simulink model "Simulink_Model"  (R2022a)
settings: Solver=VariableStepAuto  StartTime=0.0  StopTime=2474  RelTol=1e-3
values from neighbouring files (symbols this model uses):
  Air_Density = 1.2    [car__specifications.mat]
  Angle = 0    [car__specifications.mat]
  Battery_Cell_Volume = 16532.1    [car__specifications.mat]
  Battery_Cell_Weight = 0.05    [car__specifications.mat]
  constant = 0.10471975512    [car__specifications.mat]
  Drag_Coefficient = 0.2    [car__specifications.mat]
  Frontal_Area = 2.65    [car__specifications.mat]
  Gear_Ratio = 9    [car__specifications.mat]
  Motor_Efficiency = 0.95    [car__specifications.mat]
  Nominal_Battery_Cell_Current_Rating = 2.5    [car__specifications.mat]
  Nominal_Battery_Cell_Voltage = 3.6    [car__specifications.mat]
  Nominal_Battery_Pack_Voltage = 220    [car__specifications.mat]
  Range = 300    [car__specifications.mat]
  Rolling_Resistance_Coefficient = 0.02    [car__specifications.mat]
  Transmission_Efficiency = 0.8    [car__specifications.mat]
  Vehicle_Mass = 1000    [car__specifications.mat]
  Wheel_Radius = 0.3    [car__specifications.mat]
libraries: autolibshared x1
settings Model: Creator=jamesbond  LastModifiedBy=jamesbond

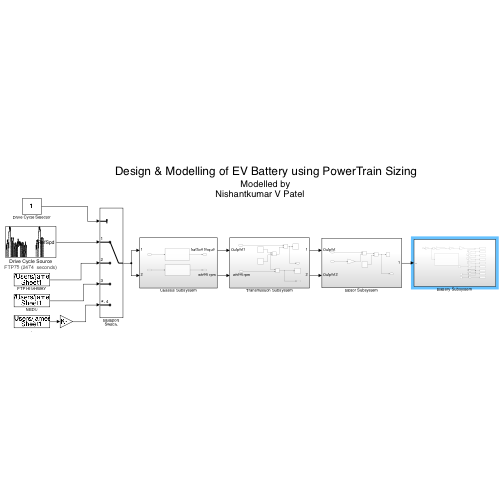
[thumbnail: Simulink's stored preview of the top-level diagram]
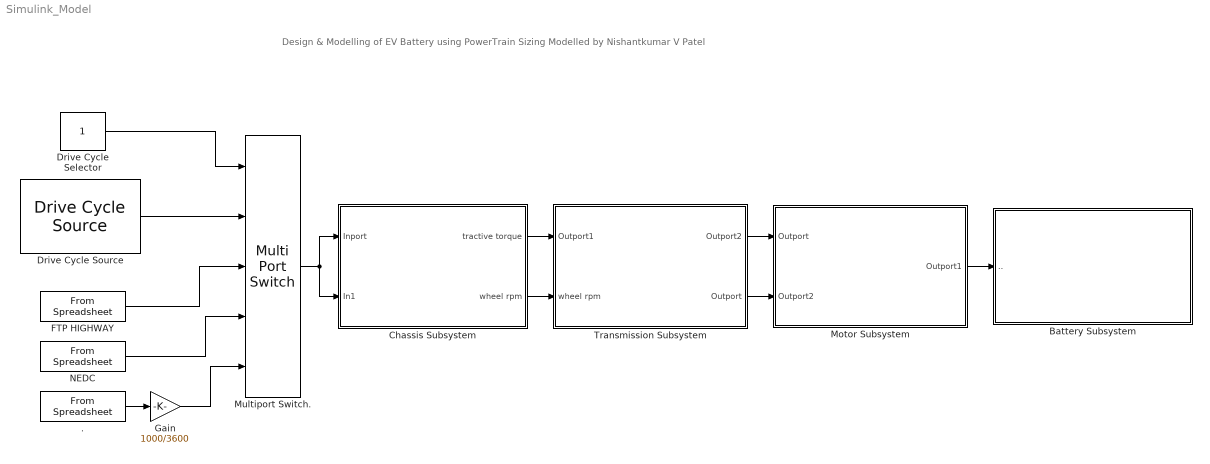
== system Simulink_Model ==
  note: Design & Modelling of EV Battery using PowerTrain Sizing
      | Modelled by
      | Nishantkumar V Patel
  . : FromSpreadsheet  FileName=/Users/jamesbond/Desktop/Mathematical Modelling of Physical Systems/Modelling & Designing EV Battery using PowerTrain Sizing Calculations /Drive Cycle Excel Files/WLTP.xlsx
  Battery Subsystem : Subsystem
  Chassis Subsystem : Subsystem
  Drive Cycle Selector : Constant
  Drive Cycle Source : autolibshared/Drive Cycle Source  cycleVar=FTP75  fileVar=WLTP.xlss  tfinal="2474  seconds"  cycleRepeat=off  outAccPort=off  outGearPort=off  gearList=No gear data  t_wot1=5  xdot_woto=0  xdot_wot1=30  t_wot2=20  xdot_wot2=0  t_wotend=30  srcUnit=m/s  outUnit=m/s  srcAccUnit=m/s/s  outAccUnit=m/s^2  dt=0  aMode=1  faultOption=off  velBnd=2  velBndUnit=mph  inUnit=m/s  timeBnd=1  failOption=off  stopSim=off  maxFaultCnt=10  maxFaultTime=2  maxTotFaultTime=15  traceOption=off  dtTrace=1  traceWindow=10  lastDCname=FTP75  lastOutUnit=mph  lastDT=0  lastTB=1  lastSB=2  forceCalcBound=off
      settings: SourceProductBaseCode=PW,DR,MT,VE
  FTP HIGHWAY : FromSpreadsheet  FileName=/Users/jamesbond/Desktop/Mathematical Modelling of Physical Systems/Modelling & Designing EV Battery using PowerTrain Sizing Calculations /Drive Cycle Excel Files/FTP_HIGHWAY.xlsx
  Gain : Gain  Gain=1000/3600
  Motor Subsystem : Subsystem
  Multiport Switch. : MultiPortSwitch  Inputs=4  SaturateOnIntegerOverflow=off  InputSameDT=off
  NEDC : FromSpreadsheet  FileName=/Users/jamesbond/Desktop/Mathematical Modelling of Physical Systems/Modelling & Designing EV Battery using PowerTrain Sizing Calculations /Drive Cycle Excel Files/NEDC.xlsx
  Transmission Subsystem : Subsystem
  wires:
  Drive Cycle Selector/1 -> Multiport Switch./1
  Drive Cycle Source/1 -> Multiport Switch./2
  FTP HIGHWAY/1 -> Multiport Switch./3
  NEDC/1 -> Multiport Switch./4
  ./1 -> Gain/1
  Gain/1 -> Multiport Switch./5
  Multiport Switch./1 -> Chassis Subsystem/1(Inport), Chassis Subsystem/2(In1)
  Motor Subsystem/1(Outport1) -> Battery Subsystem/1(..)
  Chassis Subsystem/2("  wheel rpm") -> Transmission Subsystem/2("  wheel rpm")
  Chassis Subsystem/1("tractive torque ") -> Transmission Subsystem/1(Outport1)
  Transmission Subsystem/1(Outport2) -> Motor Subsystem/1(Outport)
  Transmission Subsystem/2(Outport) -> Motor Subsystem/2(Outport2)

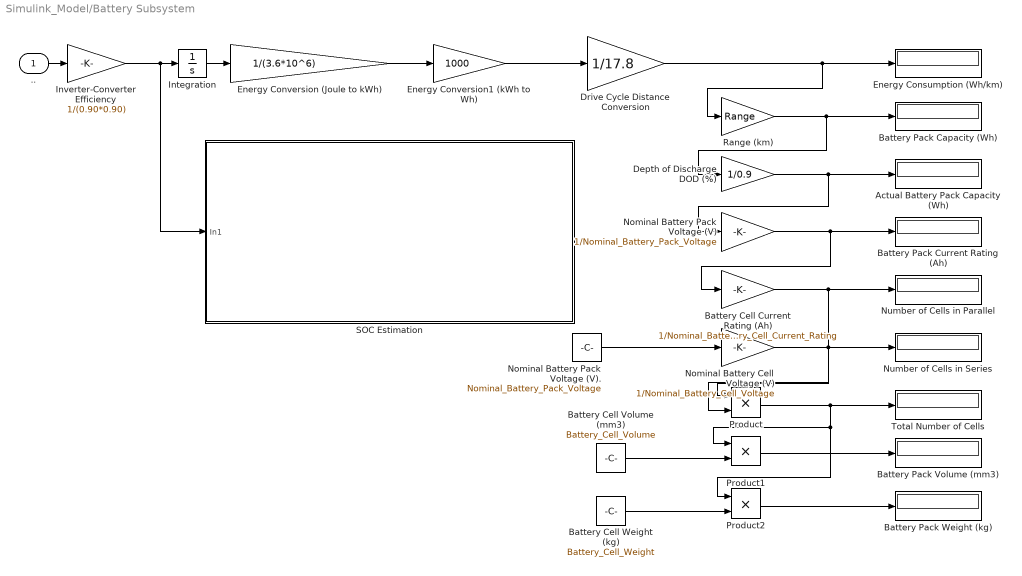
== system Simulink_Model/Battery Subsystem ==
  .. : Inport
  Actual Battery Pack Capacity (Wh) : Display
  Battery Cell Current Rating (Ah) : Gain  Gain=1/Nominal_Battery_Cell_Current_Rating
  Battery Cell Volume (mm3) : Constant  Value=Battery_Cell_Volume
  Battery Cell Weight (kg) : Constant  Value=Battery_Cell_Weight
  Battery Pack Capacity (Wh) : Display
  Battery Pack Current Rating (Ah) : Display
  Battery Pack Volume (mm3) : Display
  Battery Pack Weight (kg) : Display
  Depth of Discharge DOD (%) : Gain  Gain=1/0.9
  Drive Cycle Distance Conversion : Gain  Gain=1/17.8
  Energy Consumption (Wh/km) : Display
  "Energy Conversion (Joule to kWh) " : Gain  Gain=1/(3.6*10^6)
  Energy Conversion1 (kWh to Wh) : Gain  Gain=1000
  Integration : Integrator
  Inverter-Converter Efficiency : Gain  Gain=1/(0.90*0.90)
  Nominal Battery Cell Voltage (V) : Gain  Gain=1/Nominal_Battery_Cell_Voltage
  Nominal Battery Pack Voltage (V) : Gain  Gain=1/Nominal_Battery_Pack_Voltage
  Nominal Battery Pack Voltage (V). : Constant  Value=Nominal_Battery_Pack_Voltage
  Number of Cells in Parallel : Display
  Number of Cells in Series : Display
  Product : Product
  Product1 : Product
  Product2 : Product
  Range (km) : Gain  Gain=Range
  SOC Estimation : Subsystem
  Total Number of Cells : Display
  wires:
  ../1 -> Inverter-Converter Efficiency/1
  Inverter-Converter Efficiency/1 -> SOC Estimation/1(In1), Integration/1
  Integration/1 -> "Energy Conversion (Joule to kWh) "/1
  "Energy Conversion (Joule to kWh) "/1 -> Energy Conversion1 (kWh to Wh)/1
  Energy Conversion1 (kWh to Wh)/1 -> Drive Cycle Distance Conversion/1
  Drive Cycle Distance Conversion/1 -> Energy Consumption (Wh/km)/1, Range (km)/1
  Range (km)/1 -> Battery Pack Capacity (Wh)/1, Depth of Discharge DOD (%)/1
  Depth of Discharge DOD (%)/1 -> Actual Battery Pack Capacity (Wh)/1, Nominal Battery Pack Voltage (V)/1
  Nominal Battery Pack Voltage (V)/1 -> Battery Cell Current Rating (Ah)/1, Battery Pack Current Rating (Ah)/1
  Battery Cell Current Rating (Ah)/1 -> Number of Cells in Parallel/1, Product/1
  Nominal Battery Pack Voltage (V)./1 -> Nominal Battery Cell Voltage (V)/1
  Nominal Battery Cell Voltage (V)/1 -> Number of Cells in Series/1, Product/2
  Product/1 -> Product1/1, Product2/1, Total Number of Cells/1
  Product1/1 -> Battery Pack Volume (mm3)/1
  Battery Cell Volume (mm3)/1 -> Product1/2
  Product2/1 -> Battery Pack Weight (kg)/1
  Battery Cell Weight (kg)/1 -> Product2/2

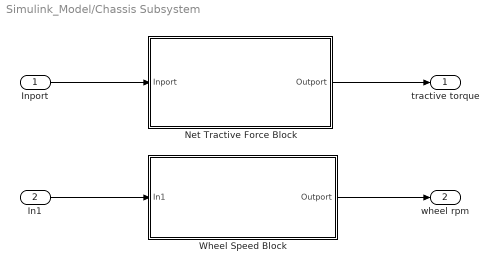
== system Simulink_Model/Chassis Subsystem ==
  Inport : Inport
  In1 : Inport  Port=2
  Net Tractive Force Block : Subsystem
  Wheel Speed Block : Subsystem
  "tractive torque " : Outport
  "  wheel rpm" : Outport  Port=2
  wires:
  Net Tractive Force Block/1(Outport) -> "tractive torque "/1
  Inport/1 -> Net Tractive Force Block/1(Inport)
  In1/1 -> Wheel Speed Block/1(In1)
  Wheel Speed Block/1(Outport) -> "  wheel rpm"/1

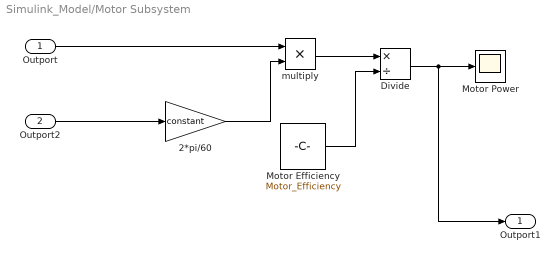
== system Simulink_Model/Motor Subsystem ==
  Outport : Inport
  Outport2 : Inport  Port=2
  2*pi/60 : Gain  Gain=constant
  Divide : Product  Inputs=*/
  Motor Efficiency : Constant  Value=Motor_Efficiency
  Motor Power : Scope
  multiply : Product
  Outport1 : Outport
  wires:
  Outport/1 -> multiply/1
  multiply/1 -> Divide/1
  Motor Efficiency/1 -> Divide/2
  2*pi/60/1 -> multiply/2
  Outport2/1 -> 2*pi/60/1
  Divide/1 -> Outport1/1, Motor Power/1

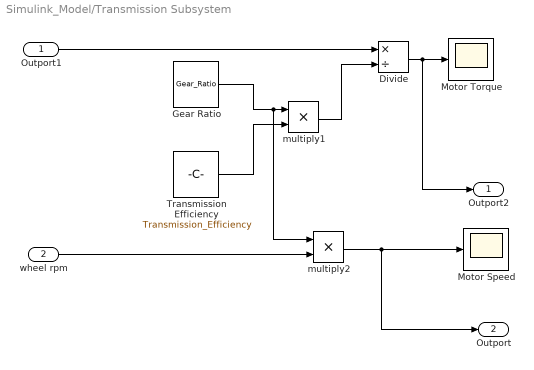
== system Simulink_Model/Transmission Subsystem ==
  Outport1 : Inport
  "  wheel rpm" : Inport  Port=2
  Divide : Product  Inputs=*/
  Gear Ratio : Constant  Value=Gear_Ratio
  Motor Speed : Scope
  Motor Torque : Scope
  Transmission Efficiency : Constant  Value=Transmission_Efficiency
  multiply1 : Product
  multiply2 : Product
  Outport2 : Outport
  Outport : Outport  Port=2
  wires:
  "  wheel rpm"/1 -> multiply2/2
  Divide/1 -> Outport2/1, Motor Torque/1
  multiply2/1 -> Outport/1, Motor Speed/1
  multiply1/1 -> Divide/2
  Outport1/1 -> Divide/1
  Transmission Efficiency/1 -> multiply1/2
  Gear Ratio/1 -> multiply2/1, multiply1/1

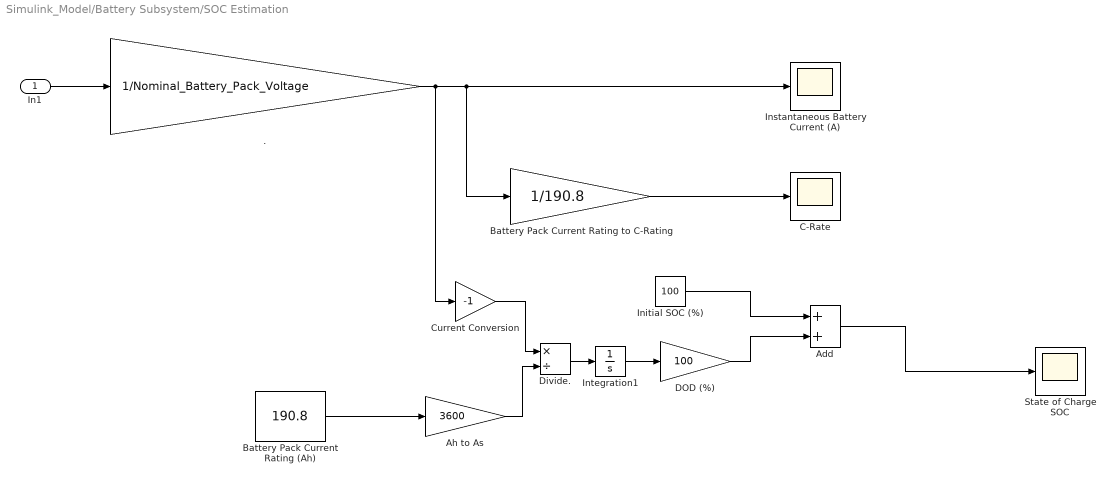
== system Simulink_Model/Battery Subsystem/SOC Estimation ==
  In1 : Inport
  . : Gain  Gain=1/Nominal_Battery_Pack_Voltage
  Add : Sum
  Ah to As : Gain  Gain=3600
  "Battery Pack Current Rating (Ah) " : Constant  Value=190.8
  Battery Pack Current Rating to C-Rating : Gain  Gain=1/190.8
  C-Rate : Scope
  Current Conversion : Gain  Gain=-1
  DOD (%) : Gain  Gain=100
  "Divide. " : Product  Inputs=*/
  Initial SOC (%) : Constant  Value=100
  Instantaneous Battery Current (A) : Scope
  Integration1 : Integrator
  State of Charge SOC : Scope
  wires:
  Add/1 -> State of Charge SOC/1
  "Battery Pack Current Rating (Ah) "/1 -> Ah to As/1
  DOD (%)/1 -> Add/2
  Current Conversion/1 -> "Divide. "/1
  "Divide. "/1 -> Integration1/1
  Initial SOC (%)/1 -> Add/1
  Integration1/1 -> DOD (%)/1
  ./1 -> Current Conversion/1, Battery Pack Current Rating to C-Rating/1, Instantaneous Battery Current (A)/1
  Battery Pack Current Rating to C-Rating/1 -> C-Rate/1
  In1/1 -> ./1
  Ah to As/1 -> "Divide. "/2

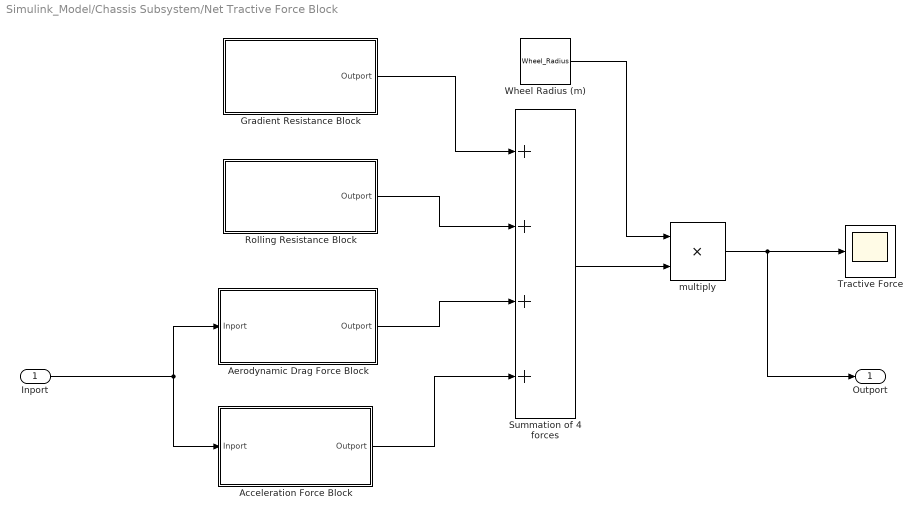
== system Simulink_Model/Chassis Subsystem/Net Tractive Force Block ==
  Inport : Inport
  Acceleration Force Block : Subsystem
  Aerodynamic Drag Force Block : Subsystem
  Gradient Resistance Block : Subsystem
  Rolling Resistance Block : Subsystem
  Summation of 4 forces : Sum  Inputs=++++
  Tractive Force : Scope
  Wheel Radius (m) : Constant  Value=Wheel_Radius
  multiply : Product
  Outport : Outport
  wires:
  Inport/1 -> Acceleration Force Block/1(Inport), Aerodynamic Drag Force Block/1(Inport)
  Gradient Resistance Block/1(Outport) -> Summation of 4 forces/1
  Aerodynamic Drag Force Block/1(Outport) -> Summation of 4 forces/3
  Rolling Resistance Block/1(Outport) -> Summation of 4 forces/2
  Acceleration Force Block/1(Outport) -> Summation of 4 forces/4
  Summation of 4 forces/1 -> multiply/2
  Wheel Radius (m)/1 -> multiply/1
  multiply/1 -> Tractive Force/1, Outport/1

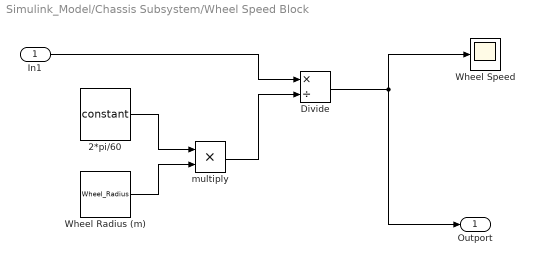
== system Simulink_Model/Chassis Subsystem/Wheel Speed Block ==
  In1 : Inport
  2*pi/60 : Constant  Value=constant
  Divide : Product  Inputs=*/
  Wheel Radius (m) : Constant  Value=Wheel_Radius
  Wheel Speed : Scope
  multiply : Product
  Outport : Outport
  wires:
  In1/1 -> Divide/1
  Wheel Radius (m)/1 -> multiply/2
  2*pi/60/1 -> multiply/1
  Divide/1 -> Wheel Speed/1, Outport/1
  multiply/1 -> Divide/2

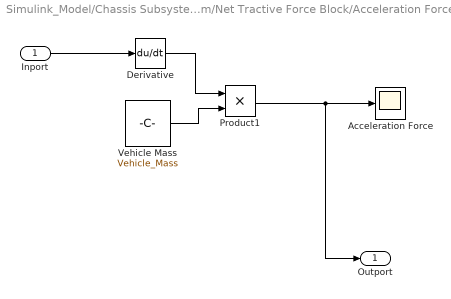
== system Simulink_Model/Chassis Subsystem/Net Tractive Force Block/Acceleration Force Block ==
  Inport : Inport
  Acceleration Force : Scope
  Derivative : Derivative
  Product1 : Product
  Vehicle Mass : Constant  Value=Vehicle_Mass
  Outport : Outport
  wires:
  Vehicle Mass/1 -> Product1/2
  Inport/1 -> Derivative/1
  Derivative/1 -> Product1/1
  Product1/1 -> Outport/1, Acceleration Force/1

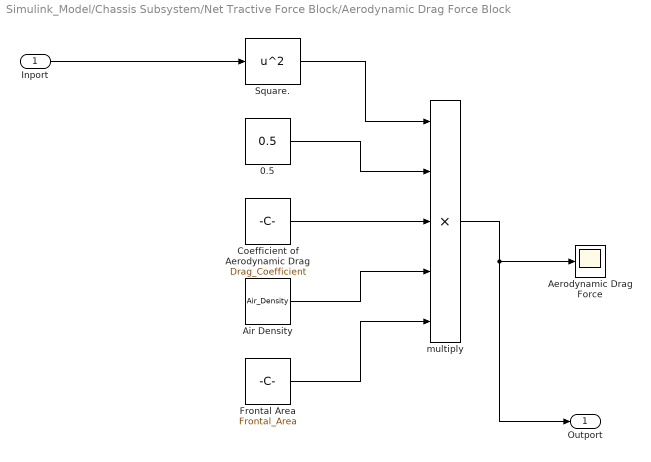
== system Simulink_Model/Chassis Subsystem/Net Tractive Force Block/Aerodynamic Drag Force Block ==
  Inport : Inport
  0.5 : Constant  Value=0.5
  Aerodynamic Drag Force : Scope
  Air Density : Constant  Value=Air_Density
  Coefficient of Aerodynamic Drag : Constant  Value=Drag_Coefficient
  Frontal Area : Constant  Value=Frontal_Area
  Square. : Math  Operator=square
  multiply : Product  Inputs=5
  Outport : Outport
  wires:
  multiply/1 -> Outport/1, Aerodynamic Drag Force/1
  Square./1 -> multiply/1
  0.5/1 -> multiply/2
  Coefficient of Aerodynamic Drag/1 -> multiply/3
  Air Density/1 -> multiply/4
  Frontal Area/1 -> multiply/5
  Inport/1 -> Square./1

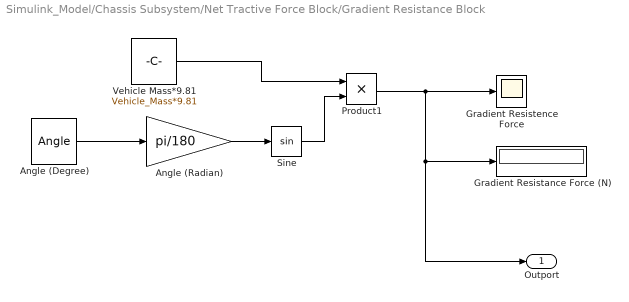
== system Simulink_Model/Chassis Subsystem/Net Tractive Force Block/Gradient Resistance Block ==
  Angle (Degree) : Constant  Value=Angle
  Angle (Radian) : Gain  Gain=pi/180
  Gradient Resistance Force (N) : Display
  Gradient Resistence Force : Scope
  Product1 : Product
  Sine : Trigonometry
  Vehicle Mass*9.81 : Constant  Value=Vehicle_Mass*9.81
  Outport : Outport
  wires:
  Angle (Radian)/1 -> Sine/1
  Sine/1 -> Product1/2
  Vehicle Mass*9.81/1 -> Product1/1
  Product1/1 -> Gradient Resistance Force (N)/1, Outport/1, Gradient Resistence Force/1
  Angle (Degree)/1 -> Angle (Radian)/1

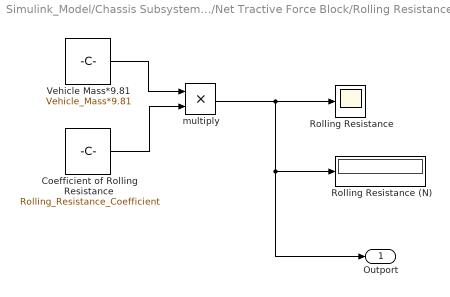
== system Simulink_Model/Chassis Subsystem/Net Tractive Force Block/Rolling Resistance Block ==
  Coefficient of Rolling Resistance : Constant  Value=Rolling_Resistance_Coefficient
  Rolling Resistance : Scope
  Rolling Resistance (N) : Display
  Vehicle Mass*9.81 : Constant  Value=Vehicle_Mass*9.81
  multiply : Product
  Outport : Outport
  wires:
  Vehicle Mass*9.81/1 -> multiply/1
  Coefficient of Rolling Resistance/1 -> multiply/2
  multiply/1 -> Rolling Resistance/1, Rolling Resistance (N)/1, Outport/1
